simulink model "RL_sus_quarter_sim"  (R2025a)
settings: Solver=FixedStepAuto  StartTime=0.0  StopTime=20  FixedStep=0.001  RelTol=1e-3
model workspace (MAT data in the model file):
  G0 : Simulink.Parameter (value not decoded)
  Q_F : Simulink.Parameter (value not decoded)
  Q_dot_s : Simulink.Parameter (value not decoded)
  Q_dot_s_h : Simulink.Parameter (value not decoded)
  Q_dot_u : Simulink.Parameter (value not decoded)
  Q_flec : Simulink.Parameter (value not decoded)
  Q_flec_t : Simulink.Parameter (value not decoded)
  b_deflec : Simulink.Parameter (value not decoded)
  bump_height : Simulink.Parameter (value not decoded)
  bump_lenth : Simulink.Parameter (value not decoded)
  bump_start : Simulink.Parameter (value not decoded)
  f0 : Simulink.Parameter (value not decoded)
  kt : Simulink.Parameter (value not decoded)
  ms : Simulink.Parameter (value not decoded)
  n0 : Simulink.Parameter (value not decoded)
  n1 : Simulink.Parameter (value not decoded)
  omega_1 : Simulink.Parameter (value not decoded)
  omega_2 : Simulink.Parameter (value not decoded)
  omega_3 : Simulink.Parameter (value not decoded)
  omega_4 : Simulink.Parameter (value not decoded)
  ramp_height : Simulink.Parameter (value not decoded)
  ramp_lenth : Simulink.Parameter (value not decoded)
  ramp_start : Simulink.Parameter (value not decoded)
  sine_amp : Simulink.Parameter (value not decoded)
  sine_freq : Simulink.Parameter (value not decoded)
  u : Simulink.Parameter (value not decoded)
symbols that are objects in the model workspace (value not decoded): b_deflec, bump_height, bump_lenth, bump_start, f0, G0, kt, ms, n0, n1, omega_1, omega_2, omega_3, omega_4, Q_dot_s, Q_dot_s_h, Q_F, Q_flec, Q_flec_t, ramp_height, ramp_lenth, ramp_start, sine_amp, sine_freq
undefined symbols (not defined in the file): Ground, Hook, SH_ADD_new_as_as_xdef
libraries: fl_lib x250, nesl_utility x48, sharedTrackingLibrary x34, dspstat3 x18, simulink x3, deeplib x2, slpidlib x1
(part 9 of 12)

== system RL_sus_quarter_sim/Quarter_sys/Control/Y_1/Freq_imp/Low_with_Alpha/Subsystem/p1_k5 ==
  Translational Inerter : fl_lib/Mechanical/Translational Elements/Translational Inerter  B=1 kg  v_specify=off  v_priority=High  v=0 m/s  v_nominal_specify=off  v_nominal_value=1  v_nominal_unit=m/s  f_specify=off  f_priority=None  f=0 N  f_nominal_specify=off  f_nominal_value=1  f_nominal_unit=N
      settings: InternalSimscapePortConfiguration="{\"Bottom\":[],\"Left\":[{\"id\":\"R\",\"label\":\"R\",\"type\":\"foundation.mechanical.translational.translational\"}],\"Right\":[{\"id\":\"C\",\"label\":\"C\",\"type\":\"foundation.mechanical.translational.translational\"}],\"Top\":[]}"
  Translational Damper : fl_lib/Mechanical/Translational Elements/Translational Damper  D=2000 N*s/m  v_specify=off  v_priority=None  v=0 m/s  v_nominal_specify=off  v_nominal_value=1  v_nominal_unit=m/s  f_specify=off  f_priority=None  f=0 N  f_nominal_specify=off  f_nominal_value=1  f_nominal_unit=N
  Translational Spring1 : fl_lib/Mechanical/Translational Elements/Translational Spring  spr_rate=20000 N/m  v_specify=off  v_priority=None  v=0 m/s  v_nominal_specify=off  v_nominal_value=1  v_nominal_unit=m/s  f_specify=off  f_priority=None  f=0 N  f_nominal_specify=off  f_nominal_value=1  f_nominal_unit=N  x_specify=off  x_priority=High  x=0 m  x_nominal_specify=off  x_nominal_value=1  x_nominal_unit=m
  Conn1 : PMIOPort  Side=Right
  Conn2 : PMIOPort  Port=2  Side=Left
  connections:
  Translational Damper/LConn1 -- Conn2/RConn1 -- Translational Inerter/LConn1
  Translational Damper/RConn1 -- Translational Spring1/LConn1 -- Translational Inerter/RConn1
  Translational Spring1/RConn1 -- Conn1/RConn1

== system RL_sus_quarter_sim/Quarter_sys/Control/Y_1/Freq_imp/Low_with_Alpha/Subsystem/passive ==
  Translational Damper : fl_lib/Mechanical/Translational Elements/Translational Damper  D=2000 N*s/m  v_specify=off  v_priority=None  v=0 m/s  v_nominal_specify=off  v_nominal_value=1  v_nominal_unit=m/s  f_specify=off  f_priority=None  f=0 N  f_nominal_specify=off  f_nominal_value=1  f_nominal_unit=N
  Translational Spring1 : fl_lib/Mechanical/Translational Elements/Translational Spring  spr_rate=200000 N/m  v_specify=off  v_priority=None  v=0 m/s  v_nominal_specify=off  v_nominal_value=1  v_nominal_unit=m/s  f_specify=off  f_priority=None  f=0 N  f_nominal_specify=off  f_nominal_value=1  f_nominal_unit=N  x_specify=off  x_priority=High  x=0 m  x_nominal_specify=off  x_nominal_value=1  x_nominal_unit=m
  Conn1 : PMIOPort  Side=Right
  Conn2 : PMIOPort  Port=2  Side=Left
  connections:
  Translational Damper/RConn1 -- Translational Spring1/RConn1 -- Conn1/RConn1
  Conn2/RConn1 -- Translational Damper/LConn1 -- Translational Spring1/LConn1

== system RL_sus_quarter_sim/Quarter_sys/Control/Y_1/Freq_imp/high_with_Alpha/Subsystem/p1_k1 ==
  Translational Inerter : fl_lib/Mechanical/Translational Elements/Translational Inerter  B=1 kg  v_specify=off  v_priority=High  v=0 m/s  v_nominal_specify=off  v_nominal_value=1  v_nominal_unit=m/s  f_specify=off  f_priority=None  f=0 N  f_nominal_specify=off  f_nominal_value=1  f_nominal_unit=N
      settings: InternalSimscapePortConfiguration="{\"Bottom\":[],\"Left\":[{\"id\":\"R\",\"label\":\"R\",\"type\":\"foundation.mechanical.translational.translational\"}],\"Right\":[{\"id\":\"C\",\"label\":\"C\",\"type\":\"foundation.mechanical.translational.translational\"}],\"Top\":[]}"
  Translational Damper : fl_lib/Mechanical/Translational Elements/Translational Damper  D=2000 N*s/m  v_specify=off  v_priority=None  v=0 m/s  v_nominal_specify=off  v_nominal_value=1  v_nominal_unit=m/s  f_specify=off  f_priority=None  f=0 N  f_nominal_specify=off  f_nominal_value=1  f_nominal_unit=N
  Translational Spring1 : fl_lib/Mechanical/Translational Elements/Translational Spring  spr_rate=20000 N/m  v_specify=off  v_priority=None  v=0 m/s  v_nominal_specify=off  v_nominal_value=1  v_nominal_unit=m/s  f_specify=off  f_priority=None  f=0 N  f_nominal_specify=off  f_nominal_value=1  f_nominal_unit=N  x_specify=off  x_priority=High  x=0 m  x_nominal_specify=off  x_nominal_value=1  x_nominal_unit=m
  Conn1 : PMIOPort  Side=Right
  Conn2 : PMIOPort  Port=2  Side=Left
  connections:
  Conn1/RConn1 -- Translational Damper/RConn1 -- Translational Spring1/RConn1
  Translational Spring1/LConn1 -- Translational Inerter/RConn1
  Conn2/RConn1 -- Translational Damper/LConn1 -- Translational Inerter/LConn1

== system RL_sus_quarter_sim/Quarter_sys/Control/Y_1/Freq_imp/high_with_Alpha/Subsystem/p1_k2 ==
  Translational Inerter : fl_lib/Mechanical/Translational Elements/Translational Inerter  B=1 kg  v_specify=off  v_priority=High  v=0 m/s  v_nominal_specify=off  v_nominal_value=1  v_nominal_unit=m/s  f_specify=off  f_priority=None  f=0 N  f_nominal_specify=off  f_nominal_value=1  f_nominal_unit=N
      settings: InternalSimscapePortConfiguration="{\"Bottom\":[],\"Left\":[{\"id\":\"R\",\"label\":\"R\",\"type\":\"foundation.mechanical.translational.translational\"}],\"Right\":[{\"id\":\"C\",\"label\":\"C\",\"type\":\"foundation.mechanical.translational.translational\"}],\"Top\":[]}"
  Translational Damper : fl_lib/Mechanical/Translational Elements/Translational Damper  D=2000 N*s/m  v_specify=off  v_priority=None  v=0 m/s  v_nominal_specify=off  v_nominal_value=1  v_nominal_unit=m/s  f_specify=off  f_priority=None  f=0 N  f_nominal_specify=off  f_nominal_value=1  f_nominal_unit=N
  Translational Spring1 : fl_lib/Mechanical/Translational Elements/Translational Spring  spr_rate=20000 N/m  v_specify=off  v_priority=None  v=0 m/s  v_nominal_specify=off  v_nominal_value=1  v_nominal_unit=m/s  f_specify=off  f_priority=None  f=0 N  f_nominal_specify=off  f_nominal_value=1  f_nominal_unit=N  x_specify=off  x_priority=High  x=0 m  x_nominal_specify=off  x_nominal_value=1  x_nominal_unit=m
  Conn1 : PMIOPort  Side=Right
  Conn2 : PMIOPort  Port=2  Side=Left
  connections:
  Translational Inerter/LConn1 -- Translational Damper/LConn1 -- Conn2/RConn1
  Translational Spring1/RConn1 -- Translational Inerter/RConn1 -- Conn1/RConn1
  Translational Spring1/LConn1 -- Translational Damper/RConn1

== system RL_sus_quarter_sim/Quarter_sys/Control/Y_1/Freq_imp/high_with_Alpha/Subsystem/p1_k3 ==
  Translational Inerter : fl_lib/Mechanical/Translational Elements/Translational Inerter  B=1 kg  v_specify=off  v_priority=High  v=0 m/s  v_nominal_specify=off  v_nominal_value=1  v_nominal_unit=m/s  f_specify=off  f_priority=None  f=0 N  f_nominal_specify=off  f_nominal_value=1  f_nominal_unit=N
      settings: InternalSimscapePortConfiguration="{\"Bottom\":[],\"Left\":[{\"id\":\"R\",\"label\":\"R\",\"type\":\"foundation.mechanical.translational.translational\"}],\"Right\":[{\"id\":\"C\",\"label\":\"C\",\"type\":\"foundation.mechanical.translational.translational\"}],\"Top\":[]}"
  Translational Damper : fl_lib/Mechanical/Translational Elements/Translational Damper  D=2000 N*s/m  v_specify=off  v_priority=None  v=0 m/s  v_nominal_specify=off  v_nominal_value=1  v_nominal_unit=m/s  f_specify=off  f_priority=None  f=0 N  f_nominal_specify=off  f_nominal_value=1  f_nominal_unit=N
  Translational Spring1 : fl_lib/Mechanical/Translational Elements/Translational Spring  spr_rate=20000 N/m  v_specify=off  v_priority=None  v=0 m/s  v_nominal_specify=off  v_nominal_value=1  v_nominal_unit=m/s  f_specify=off  f_priority=None  f=0 N  f_nominal_specify=off  f_nominal_value=1  f_nominal_unit=N  x_specify=off  x_priority=High  x=0 m  x_nominal_specify=off  x_nominal_value=1  x_nominal_unit=m
  Conn1 : PMIOPort  Side=Right
  Conn2 : PMIOPort  Port=2  Side=Left
  connections:
  Conn2/RConn1 -- Translational Damper/LConn1 -- Translational Inerter/LConn1 -- Translational Spring1/LConn1
  Translational Inerter/RConn1 -- Conn1/RConn1 -- Translational Damper/RConn1 -- Translational Spring1/RConn1

== system RL_sus_quarter_sim/Quarter_sys/Control/Y_1/Freq_imp/high_with_Alpha/Subsystem/p1_k5 ==
  Translational Inerter : fl_lib/Mechanical/Translational Elements/Translational Inerter  B=1 kg  v_specify=off  v_priority=High  v=0 m/s  v_nominal_specify=off  v_nominal_value=1  v_nominal_unit=m/s  f_specify=off  f_priority=None  f=0 N  f_nominal_specify=off  f_nominal_value=1  f_nominal_unit=N
      settings: InternalSimscapePortConfiguration="{\"Bottom\":[],\"Left\":[{\"id\":\"R\",\"label\":\"R\",\"type\":\"foundation.mechanical.translational.translational\"}],\"Right\":[{\"id\":\"C\",\"label\":\"C\",\"type\":\"foundation.mechanical.translational.translational\"}],\"Top\":[]}"
  Translational Damper : fl_lib/Mechanical/Translational Elements/Translational Damper  D=2000 N*s/m  v_specify=off  v_priority=None  v=0 m/s  v_nominal_specify=off  v_nominal_value=1  v_nominal_unit=m/s  f_specify=off  f_priority=None  f=0 N  f_nominal_specify=off  f_nominal_value=1  f_nominal_unit=N
  Translational Spring1 : fl_lib/Mechanical/Translational Elements/Translational Spring  spr_rate=20000 N/m  v_specify=off  v_priority=None  v=0 m/s  v_nominal_specify=off  v_nominal_value=1  v_nominal_unit=m/s  f_specify=off  f_priority=None  f=0 N  f_nominal_specify=off  f_nominal_value=1  f_nominal_unit=N  x_specify=off  x_priority=High  x=0 m  x_nominal_specify=off  x_nominal_value=1  x_nominal_unit=m
  Conn1 : PMIOPort  Side=Right
  Conn2 : PMIOPort  Port=2  Side=Left
  connections:
  Translational Spring1/RConn1 -- Conn1/RConn1
  Translational Inerter/RConn1 -- Translational Spring1/LConn1 -- Translational Damper/RConn1
  Translational Inerter/LConn1 -- Conn2/RConn1 -- Translational Damper/LConn1

== system RL_sus_quarter_sim/Quarter_sys/Control/Y_1/Freq_imp/high_with_Alpha/Subsystem/passive ==
  Translational Damper : fl_lib/Mechanical/Translational Elements/Translational Damper  D=2000 N*s/m  v_specify=off  v_priority=None  v=0 m/s  v_nominal_specify=off  v_nominal_value=1  v_nominal_unit=m/s  f_specify=off  f_priority=None  f=0 N  f_nominal_specify=off  f_nominal_value=1  f_nominal_unit=N
  Translational Spring1 : fl_lib/Mechanical/Translational Elements/Translational Spring  spr_rate=200000 N/m  v_specify=off  v_priority=None  v=0 m/s  v_nominal_specify=off  v_nominal_value=1  v_nominal_unit=m/s  f_specify=off  f_priority=None  f=0 N  f_nominal_specify=off  f_nominal_value=1  f_nominal_unit=N  x_specify=off  x_priority=High  x=0 m  x_nominal_specify=off  x_nominal_value=1  x_nominal_unit=m
  Conn1 : PMIOPort  Side=Right
  Conn2 : PMIOPort  Port=2  Side=Left
  connections:
  Translational Spring1/LConn1 -- Translational Damper/LConn1 -- Conn2/RConn1
  Conn1/RConn1 -- Translational Spring1/RConn1 -- Translational Damper/RConn1

== system RL_sus_quarter_sim/Quarter_sys/Control/Y_1/Freq_imp1/Low_with_Alpha/Subsystem/p1_k1 ==
  Translational Inerter : fl_lib/Mechanical/Translational Elements/Translational Inerter  B=1 kg  v_specify=off  v_priority=High  v=0 m/s  v_nominal_specify=off  v_nominal_value=1  v_nominal_unit=m/s  f_specify=off  f_priority=None  f=0 N  f_nominal_specify=off  f_nominal_value=1  f_nominal_unit=N
      settings: InternalSimscapePortConfiguration="{\"Bottom\":[],\"Left\":[{\"id\":\"R\",\"label\":\"R\",\"type\":\"foundation.mechanical.translational.translational\"}],\"Right\":[{\"id\":\"C\",\"label\":\"C\",\"type\":\"foundation.mechanical.translational.translational\"}],\"Top\":[]}"
  Translational Damper : fl_lib/Mechanical/Translational Elements/Translational Damper  D=2000 N*s/m  v_specify=off  v_priority=None  v=0 m/s  v_nominal_specify=off  v_nominal_value=1  v_nominal_unit=m/s  f_specify=off  f_priority=None  f=0 N  f_nominal_specify=off  f_nominal_value=1  f_nominal_unit=N
  Translational Spring1 : fl_lib/Mechanical/Translational Elements/Translational Spring  spr_rate=20000 N/m  v_specify=off  v_priority=None  v=0 m/s  v_nominal_specify=off  v_nominal_value=1  v_nominal_unit=m/s  f_specify=off  f_priority=None  f=0 N  f_nominal_specify=off  f_nominal_value=1  f_nominal_unit=N  x_specify=off  x_priority=High  x=0 m  x_nominal_specify=off  x_nominal_value=1  x_nominal_unit=m
  Conn1 : PMIOPort  Side=Right
  Conn2 : PMIOPort  Port=2  Side=Left
  connections:
  Conn1/RConn1 -- Translational Damper/RConn1 -- Translational Spring1/RConn1
  Translational Spring1/LConn1 -- Translational Inerter/RConn1
  Conn2/RConn1 -- Translational Damper/LConn1 -- Translational Inerter/LConn1

== system RL_sus_quarter_sim/Quarter_sys/Control/Y_1/Freq_imp1/Low_with_Alpha/Subsystem/p1_k2 ==
  Translational Inerter : fl_lib/Mechanical/Translational Elements/Translational Inerter  B=1 kg  v_specify=off  v_priority=High  v=0 m/s  v_nominal_specify=off  v_nominal_value=1  v_nominal_unit=m/s  f_specify=off  f_priority=None  f=0 N  f_nominal_specify=off  f_nominal_value=1  f_nominal_unit=N
      settings: InternalSimscapePortConfiguration="{\"Bottom\":[],\"Left\":[{\"id\":\"R\",\"label\":\"R\",\"type\":\"foundation.mechanical.translational.translational\"}],\"Right\":[{\"id\":\"C\",\"label\":\"C\",\"type\":\"foundation.mechanical.translational.translational\"}],\"Top\":[]}"
  Translational Damper : fl_lib/Mechanical/Translational Elements/Translational Damper  D=2000 N*s/m  v_specify=off  v_priority=None  v=0 m/s  v_nominal_specify=off  v_nominal_value=1  v_nominal_unit=m/s  f_specify=off  f_priority=None  f=0 N  f_nominal_specify=off  f_nominal_value=1  f_nominal_unit=N
  Translational Spring1 : fl_lib/Mechanical/Translational Elements/Translational Spring  spr_rate=20000 N/m  v_specify=off  v_priority=None  v=0 m/s  v_nominal_specify=off  v_nominal_value=1  v_nominal_unit=m/s  f_specify=off  f_priority=None  f=0 N  f_nominal_specify=off  f_nominal_value=1  f_nominal_unit=N  x_specify=off  x_priority=High  x=0 m  x_nominal_specify=off  x_nominal_value=1  x_nominal_unit=m
  Conn1 : PMIOPort  Side=Right
  Conn2 : PMIOPort  Port=2  Side=Left
  connections:
  Translational Inerter/LConn1 -- Translational Damper/LConn1 -- Conn2/RConn1
  Translational Spring1/RConn1 -- Translational Inerter/RConn1 -- Conn1/RConn1
  Translational Spring1/LConn1 -- Translational Damper/RConn1

== system RL_sus_quarter_sim/Quarter_sys/Control/Y_1/Freq_imp1/Low_with_Alpha/Subsystem/p1_k3 ==
  Translational Inerter : fl_lib/Mechanical/Translational Elements/Translational Inerter  B=1 kg  v_specify=off  v_priority=High  v=0 m/s  v_nominal_specify=off  v_nominal_value=1  v_nominal_unit=m/s  f_specify=off  f_priority=None  f=0 N  f_nominal_specify=off  f_nominal_value=1  f_nominal_unit=N
      settings: InternalSimscapePortConfiguration="{\"Bottom\":[],\"Left\":[{\"id\":\"R\",\"label\":\"R\",\"type\":\"foundation.mechanical.translational.translational\"}],\"Right\":[{\"id\":\"C\",\"label\":\"C\",\"type\":\"foundation.mechanical.translational.translational\"}],\"Top\":[]}"
  Translational Damper : fl_lib/Mechanical/Translational Elements/Translational Damper  D=2000 N*s/m  v_specify=off  v_priority=None  v=0 m/s  v_nominal_specify=off  v_nominal_value=1  v_nominal_unit=m/s  f_specify=off  f_priority=None  f=0 N  f_nominal_specify=off  f_nominal_value=1  f_nominal_unit=N
  Translational Spring1 : fl_lib/Mechanical/Translational Elements/Translational Spring  spr_rate=20000 N/m  v_specify=off  v_priority=None  v=0 m/s  v_nominal_specify=off  v_nominal_value=1  v_nominal_unit=m/s  f_specify=off  f_priority=None  f=0 N  f_nominal_specify=off  f_nominal_value=1  f_nominal_unit=N  x_specify=off  x_priority=High  x=0 m  x_nominal_specify=off  x_nominal_value=1  x_nominal_unit=m
  Conn1 : PMIOPort  Side=Right
  Conn2 : PMIOPort  Port=2  Side=Left
  connections:
  Conn2/RConn1 -- Translational Damper/LConn1 -- Translational Inerter/LConn1 -- Translational Spring1/LConn1
  Translational Inerter/RConn1 -- Conn1/RConn1 -- Translational Damper/RConn1 -- Translational Spring1/RConn1

== system RL_sus_quarter_sim/Quarter_sys/Control/Y_1/Freq_imp1/Low_with_Alpha/Subsystem/p1_k5 ==
  Translational Inerter : fl_lib/Mechanical/Translational Elements/Translational Inerter  B=1 kg  v_specify=off  v_priority=High  v=0 m/s  v_nominal_specify=off  v_nominal_value=1  v_nominal_unit=m/s  f_specify=off  f_priority=None  f=0 N  f_nominal_specify=off  f_nominal_value=1  f_nominal_unit=N
      settings: InternalSimscapePortConfiguration="{\"Bottom\":[],\"Left\":[{\"id\":\"R\",\"label\":\"R\",\"type\":\"foundation.mechanical.translational.translational\"}],\"Right\":[{\"id\":\"C\",\"label\":\"C\",\"type\":\"foundation.mechanical.translational.translational\"}],\"Top\":[]}"
  Translational Damper : fl_lib/Mechanical/Translational Elements/Translational Damper  D=2000 N*s/m  v_specify=off  v_priority=None  v=0 m/s  v_nominal_specify=off  v_nominal_value=1  v_nominal_unit=m/s  f_specify=off  f_priority=None  f=0 N  f_nominal_specify=off  f_nominal_value=1  f_nominal_unit=N
  Translational Spring1 : fl_lib/Mechanical/Translational Elements/Translational Spring  spr_rate=20000 N/m  v_specify=off  v_priority=None  v=0 m/s  v_nominal_specify=off  v_nominal_value=1  v_nominal_unit=m/s  f_specify=off  f_priority=None  f=0 N  f_nominal_specify=off  f_nominal_value=1  f_nominal_unit=N  x_specify=off  x_priority=High  x=0 m  x_nominal_specify=off  x_nominal_value=1  x_nominal_unit=m
  Conn1 : PMIOPort  Side=Right
  Conn2 : PMIOPort  Port=2  Side=Left
  connections:
  Translational Spring1/RConn1 -- Conn1/RConn1
  Translational Inerter/RConn1 -- Translational Spring1/LConn1 -- Translational Damper/RConn1
  Translational Inerter/LConn1 -- Conn2/RConn1 -- Translational Damper/LConn1

== system RL_sus_quarter_sim/Quarter_sys/Control/Y_1/Freq_imp1/Low_with_Alpha/Subsystem/passive ==
  Translational Damper : fl_lib/Mechanical/Translational Elements/Translational Damper  D=2000 N*s/m  v_specify=off  v_priority=None  v=0 m/s  v_nominal_specify=off  v_nominal_value=1  v_nominal_unit=m/s  f_specify=off  f_priority=None  f=0 N  f_nominal_specify=off  f_nominal_value=1  f_nominal_unit=N
  Translational Spring1 : fl_lib/Mechanical/Translational Elements/Translational Spring  spr_rate=200000 N/m  v_specify=off  v_priority=None  v=0 m/s  v_nominal_specify=off  v_nominal_value=1  v_nominal_unit=m/s  f_specify=off  f_priority=None  f=0 N  f_nominal_specify=off  f_nominal_value=1  f_nominal_unit=N  x_specify=off  x_priority=High  x=0 m  x_nominal_specify=off  x_nominal_value=1  x_nominal_unit=m
  Conn1 : PMIOPort  Side=Right
  Conn2 : PMIOPort  Port=2  Side=Left
  connections:
  Translational Spring1/LConn1 -- Translational Damper/LConn1 -- Conn2/RConn1
  Conn1/RConn1 -- Translational Spring1/RConn1 -- Translational Damper/RConn1

== system RL_sus_quarter_sim/Quarter_sys/Control/Y_1/Freq_imp1/high_with_Alpha/Subsystem/p1_k1 ==
  Translational Inerter : fl_lib/Mechanical/Translational Elements/Translational Inerter  B=1 kg  v_specify=off  v_priority=High  v=0 m/s  v_nominal_specify=off  v_nominal_value=1  v_nominal_unit=m/s  f_specify=off  f_priority=None  f=0 N  f_nominal_specify=off  f_nominal_value=1  f_nominal_unit=N
      settings: InternalSimscapePortConfiguration="{\"Bottom\":[],\"Left\":[{\"id\":\"R\",\"label\":\"R\",\"type\":\"foundation.mechanical.translational.translational\"}],\"Right\":[{\"id\":\"C\",\"label\":\"C\",\"type\":\"foundation.mechanical.translational.translational\"}],\"Top\":[]}"
  Translational Damper : fl_lib/Mechanical/Translational Elements/Translational Damper  D=2000 N*s/m  v_specify=off  v_priority=None  v=0 m/s  v_nominal_specify=off  v_nominal_value=1  v_nominal_unit=m/s  f_specify=off  f_priority=None  f=0 N  f_nominal_specify=off  f_nominal_value=1  f_nominal_unit=N
  Translational Spring1 : fl_lib/Mechanical/Translational Elements/Translational Spring  spr_rate=20000 N/m  v_specify=off  v_priority=None  v=0 m/s  v_nominal_specify=off  v_nominal_value=1  v_nominal_unit=m/s  f_specify=off  f_priority=None  f=0 N  f_nominal_specify=off  f_nominal_value=1  f_nominal_unit=N  x_specify=off  x_priority=High  x=0 m  x_nominal_specify=off  x_nominal_value=1  x_nominal_unit=m
  Conn1 : PMIOPort  Side=Right
  Conn2 : PMIOPort  Port=2  Side=Left
  connections:
  Translational Inerter/LConn1 -- Translational Damper/LConn1 -- Conn2/RConn1
  Translational Spring1/LConn1 -- Translational Inerter/RConn1
  Translational Spring1/RConn1 -- Translational Damper/RConn1 -- Conn1/RConn1

== system RL_sus_quarter_sim/Quarter_sys/Control/Y_1/Freq_imp1/high_with_Alpha/Subsystem/p1_k2 ==
  Translational Inerter : fl_lib/Mechanical/Translational Elements/Translational Inerter  B=1 kg  v_specify=off  v_priority=High  v=0 m/s  v_nominal_specify=off  v_nominal_value=1  v_nominal_unit=m/s  f_specify=off  f_priority=None  f=0 N  f_nominal_specify=off  f_nominal_value=1  f_nominal_unit=N
      settings: InternalSimscapePortConfiguration="{\"Bottom\":[],\"Left\":[{\"id\":\"R\",\"label\":\"R\",\"type\":\"foundation.mechanical.translational.translational\"}],\"Right\":[{\"id\":\"C\",\"label\":\"C\",\"type\":\"foundation.mechanical.translational.translational\"}],\"Top\":[]}"
  Translational Damper : fl_lib/Mechanical/Translational Elements/Translational Damper  D=2000 N*s/m  v_specify=off  v_priority=None  v=0 m/s  v_nominal_specify=off  v_nominal_value=1  v_nominal_unit=m/s  f_specify=off  f_priority=None  f=0 N  f_nominal_specify=off  f_nominal_value=1  f_nominal_unit=N
  Translational Spring1 : fl_lib/Mechanical/Translational Elements/Translational Spring  spr_rate=20000 N/m  v_specify=off  v_priority=None  v=0 m/s  v_nominal_specify=off  v_nominal_value=1  v_nominal_unit=m/s  f_specify=off  f_priority=None  f=0 N  f_nominal_specify=off  f_nominal_value=1  f_nominal_unit=N  x_specify=off  x_priority=High  x=0 m  x_nominal_specify=off  x_nominal_value=1  x_nominal_unit=m
  Conn1 : PMIOPort  Side=Right
  Conn2 : PMIOPort  Port=2  Side=Left
  connections:
  Translational Spring1/LConn1 -- Translational Damper/RConn1
  Conn1/RConn1 -- Translational Inerter/RConn1 -- Translational Spring1/RConn1
  Conn2/RConn1 -- Translational Damper/LConn1 -- Translational Inerter/LConn1

== system RL_sus_quarter_sim/Quarter_sys/Control/Y_1/Freq_imp1/high_with_Alpha/Subsystem/p1_k3 ==
  Translational Inerter : fl_lib/Mechanical/Translational Elements/Translational Inerter  B=1 kg  v_specify=off  v_priority=High  v=0 m/s  v_nominal_specify=off  v_nominal_value=1  v_nominal_unit=m/s  f_specify=off  f_priority=None  f=0 N  f_nominal_specify=off  f_nominal_value=1  f_nominal_unit=N
      settings: InternalSimscapePortConfiguration="{\"Bottom\":[],\"Left\":[{\"id\":\"R\",\"label\":\"R\",\"type\":\"foundation.mechanical.translational.translational\"}],\"Right\":[{\"id\":\"C\",\"label\":\"C\",\"type\":\"foundation.mechanical.translational.translational\"}],\"Top\":[]}"
  Translational Damper : fl_lib/Mechanical/Translational Elements/Translational Damper  D=2000 N*s/m  v_specify=off  v_priority=None  v=0 m/s  v_nominal_specify=off  v_nominal_value=1  v_nominal_unit=m/s  f_specify=off  f_priority=None  f=0 N  f_nominal_specify=off  f_nominal_value=1  f_nominal_unit=N
  Translational Spring1 : fl_lib/Mechanical/Translational Elements/Translational Spring  spr_rate=20000 N/m  v_specify=off  v_priority=None  v=0 m/s  v_nominal_specify=off  v_nominal_value=1  v_nominal_unit=m/s  f_specify=off  f_priority=None  f=0 N  f_nominal_specify=off  f_nominal_value=1  f_nominal_unit=N  x_specify=off  x_priority=High  x=0 m  x_nominal_specify=off  x_nominal_value=1  x_nominal_unit=m
  Conn1 : PMIOPort  Side=Right
  Conn2 : PMIOPort  Port=2  Side=Left
  connections:
  Translational Spring1/RConn1 -- Translational Damper/RConn1 -- Conn1/RConn1 -- Translational Inerter/RConn1
  Translational Spring1/LConn1 -- Translational Inerter/LConn1 -- Translational Damper/LConn1 -- Conn2/RConn1

== system RL_sus_quarter_sim/Quarter_sys/Control/Y_1/Freq_imp1/high_with_Alpha/Subsystem/p1_k5 ==
  Translational Inerter : fl_lib/Mechanical/Translational Elements/Translational Inerter  B=1 kg  v_specify=off  v_priority=High  v=0 m/s  v_nominal_specify=off  v_nominal_value=1  v_nominal_unit=m/s  f_specify=off  f_priority=None  f=0 N  f_nominal_specify=off  f_nominal_value=1  f_nominal_unit=N
      settings: InternalSimscapePortConfiguration="{\"Bottom\":[],\"Left\":[{\"id\":\"R\",\"label\":\"R\",\"type\":\"foundation.mechanical.translational.translational\"}],\"Right\":[{\"id\":\"C\",\"label\":\"C\",\"type\":\"foundation.mechanical.translational.translational\"}],\"Top\":[]}"
  Translational Damper : fl_lib/Mechanical/Translational Elements/Translational Damper  D=2000 N*s/m  v_specify=off  v_priority=None  v=0 m/s  v_nominal_specify=off  v_nominal_value=1  v_nominal_unit=m/s  f_specify=off  f_priority=None  f=0 N  f_nominal_specify=off  f_nominal_value=1  f_nominal_unit=N
  Translational Spring1 : fl_lib/Mechanical/Translational Elements/Translational Spring  spr_rate=20000 N/m  v_specify=off  v_priority=None  v=0 m/s  v_nominal_specify=off  v_nominal_value=1  v_nominal_unit=m/s  f_specify=off  f_priority=None  f=0 N  f_nominal_specify=off  f_nominal_value=1  f_nominal_unit=N  x_specify=off  x_priority=High  x=0 m  x_nominal_specify=off  x_nominal_value=1  x_nominal_unit=m
  Conn1 : PMIOPort  Side=Right
  Conn2 : PMIOPort  Port=2  Side=Left
  connections:
  Translational Damper/LConn1 -- Conn2/RConn1 -- Translational Inerter/LConn1
  Translational Damper/RConn1 -- Translational Spring1/LConn1 -- Translational Inerter/RConn1
  Translational Spring1/RConn1 -- Conn1/RConn1

== system RL_sus_quarter_sim/Quarter_sys/Control/Y_1/Freq_imp1/high_with_Alpha/Subsystem/passive ==
  Translational Damper : fl_lib/Mechanical/Translational Elements/Translational Damper  D=2000 N*s/m  v_specify=off  v_priority=None  v=0 m/s  v_nominal_specify=off  v_nominal_value=1  v_nominal_unit=m/s  f_specify=off  f_priority=None  f=0 N  f_nominal_specify=off  f_nominal_value=1  f_nominal_unit=N
  Translational Spring1 : fl_lib/Mechanical/Translational Elements/Translational Spring  spr_rate=200000 N/m  v_specify=off  v_priority=None  v=0 m/s  v_nominal_specify=off  v_nominal_value=1  v_nominal_unit=m/s  f_specify=off  f_priority=None  f=0 N  f_nominal_specify=off  f_nominal_value=1  f_nominal_unit=N  x_specify=off  x_priority=High  x=0 m  x_nominal_specify=off  x_nominal_value=1  x_nominal_unit=m
  Conn1 : PMIOPort  Side=Right
  Conn2 : PMIOPort  Port=2  Side=Left
  connections:
  Translational Damper/RConn1 -- Translational Spring1/RConn1 -- Conn1/RConn1
  Conn2/RConn1 -- Translational Damper/LConn1 -- Translational Spring1/LConn1

== system RL_sus_quarter_sim/Quarter_sys/Control/Y_1/IFEKF FDC/Subsystem/MATLAB Function2/EKF epsilon ==
  y : Inport
  epsilon : Inport  Port=2
  Constant : Constant  Value=diag([0,0,1,0])
  Constant7 : Constant  Value=500  SampleTime=0.001
  Extended Kalman Filter1 : sharedTrackingLibrary/Extended Kalman Filter  StateTransitionFcn=IFEKF_tfcn_ep  HasStateTransitionJacobianFcn=on  StateTransitionJacobianFcn=IFEKF_jcob_fcn_ep  HasAdditiveProcessNoise=Additive  ProcessNoise=[0,0,1e-7,1e-10]  HasTimeVaryingProcessNoise=on  HasStateTransitionFcnExtraArgument=1  InitialState=[0;-0.2;1*2*pi;0.2;]  InitialStateCovariance=[1e-1,1e-1,1e-1,1e-5]  MeasurementFcn1=IFEKF_measure_fcn_mod  HasMeasurementJacobianFcn1=on  MeasurementJacobianFcn1=IFEKF_mea_jcob_fcn_mod  HasMeasurementEnablePort1=off  HasAdditiveMeasurementNoise1=Additive  MeasurementNoise1=0.0001  HasTimeVaryingMeasurementNoise1=on  HasMeasurementFcnExtraArgument1=0  HasMeasurementWrapping1=off  MeasurementFcn2=myMeasurementFcn  HasMeasurementJacobianFcn2=off  HasMeasurementEnablePort2=off  HasAdditiveMeasurementNoise2=Additive  MeasurementNoise2=1  HasTimeVaryingMeasurementNoise2=off  HasMeasurementFcnExtraArgument2=0  HasMeasurementWrapping2=off  MeasurementFcn3=myMeasurementFcn  HasMeasurementJacobianFcn3=off  HasMeasurementEnablePort3=off  HasAdditiveMeasurementNoise3=Additive  MeasurementNoise3=1  HasTimeVaryingMeasurementNoise3=off  HasMeasurementFcnExtraArgument3=0  HasMeasurementWrapping3=off  MeasurementFcn4=myMeasurementFcn  HasMeasurementJacobianFcn4=off  HasMeasurementEnablePort4=off  HasAdditiveMeasurementNoise4=Additive  MeasurementNoise4=1  HasTimeVaryingMeasurementNoise4=off  HasMeasurementFcnExtraArgument4=0  HasMeasurementWrapping4=off  MeasurementFcn5=myMeasurementFcn  HasMeasurementJacobianFcn5=off  HasMeasurementEnablePort5=off  HasAdditiveMeasurementNoise5=Additive  MeasurementNoise5=1  HasTimeVaryingMeasurementNoise5=off  HasMeasurementFcnExtraArgument5=0  HasMeasurementWrapping5=off  EnableMultirate=off  StateTransitionFcnSampleTime=1  MeasurementFcn1SampleTime=1  MeasurementFcn2SampleTime=1  MeasurementFcn3SampleTime=1  MeasurementFcn4SampleTime=1  MeasurementFcn5SampleTime=1  UseCurrentEstimator=off  OutputStateCovariance=on  DataType=double  SampleTime=0.001  NumberOfMeasurements=1
  Gain6 : Gain  Gain=1/2/pi
  Scope6 : Scope
      settings: ActiveDisplayYMinimum=-0.3996  ActiveDisplayYMaximum=6.53697  DataLoggingVariableName=ScopeData2
  Selector1 : Selector  InputPortWidth=4  IndexOptions=Index vector (dialog)  Indices=[1]  OutputSizes=1
  Selector8 : Selector  InputPortWidth=4  IndexOptions=Index vector (dialog)  Indices=[3]  OutputSizes=1
  x1hat : Outport
  P : Outport  Port=2
  debug : Outport  Port=3
  xhat_pred : Outport  Port=4
  y_residual : Outport  Port=5
  omega : Outport  Port=6
  wires:
  y/1 -> Extended Kalman Filter1/3
  Extended Kalman Filter1/2 -> P/1
  Constant7/1 -> Extended Kalman Filter1/4
  epsilon/1 -> Extended Kalman Filter1/2
  Constant/1 -> Extended Kalman Filter1/1
  Gain6/1 -> omega/1, Scope6/1
  Selector8/1 -> Gain6/1
  Extended Kalman Filter1/1 -> Selector1/1, Selector8/1
  Selector1/1 -> x1hat/1

== system RL_sus_quarter_sim/Quarter_sys/Control/Y_1/IFEKF FDC/Subsystem/MATLAB Function2/EKF simple Amp ==
  y : Inport
  epsilon : Inport  Port=2
  Constant5 : Constant  Value=0.1e-5
  Constant7 : Constant  Value=0.11  SampleTime=0.001
  Extended Kalman Filter1 : sharedTrackingLibrary/Extended Kalman Filter  StateTransitionFcn=IFEKF_tfcn_amp  HasStateTransitionJacobianFcn=on  StateTransitionJacobianFcn=IFEKF_jcob_fcn_amp  HasAdditiveProcessNoise=Additive  ProcessNoise=[0,0,1e-7,1e-10]  HasTimeVaryingProcessNoise=on  HasStateTransitionFcnExtraArgument=1  InitialState=[0;-0.5;2*pi;0.5;]  InitialStateCovariance=[1e-1,1e-1,1e-1,1e-5]  MeasurementFcn1=IFEKF_measure_fcn_amp  HasMeasurementJacobianFcn1=on  MeasurementJacobianFcn1=IFEKF_mea_jcob_fcn_amp  HasMeasurementEnablePort1=off  HasAdditiveMeasurementNoise1=Additive  MeasurementNoise1=0.0001  HasTimeVaryingMeasurementNoise1=on  HasMeasurementFcnExtraArgument1=0  HasMeasurementWrapping1=off  MeasurementFcn2=myMeasurementFcn  HasMeasurementJacobianFcn2=off  HasMeasurementEnablePort2=off  HasAdditiveMeasurementNoise2=Additive  MeasurementNoise2=1  HasTimeVaryingMeasurementNoise2=off  HasMeasurementFcnExtraArgument2=0  HasMeasurementWrapping2=off  MeasurementFcn3=myMeasurementFcn  HasMeasurementJacobianFcn3=off  HasMeasurementEnablePort3=off  HasAdditiveMeasurementNoise3=Additive  MeasurementNoise3=1  HasTimeVaryingMeasurementNoise3=off  HasMeasurementFcnExtraArgument3=0  HasMeasurementWrapping3=off  MeasurementFcn4=myMeasurementFcn  HasMeasurementJacobianFcn4=off  HasMeasurementEnablePort4=off  HasAdditiveMeasurementNoise4=Additive  MeasurementNoise4=1  HasTimeVaryingMeasurementNoise4=off  HasMeasurementFcnExtraArgument4=0  HasMeasurementWrapping4=off  MeasurementFcn5=myMeasurementFcn  HasMeasurementJacobianFcn5=off  HasMeasurementEnablePort5=off  HasAdditiveMeasurementNoise5=Additive  MeasurementNoise5=1  HasTimeVaryingMeasurementNoise5=off  HasMeasurementFcnExtraArgument5=0  HasMeasurementWrapping5=off  EnableMultirate=off  StateTransitionFcnSampleTime=1  MeasurementFcn1SampleTime=1  MeasurementFcn2SampleTime=1  MeasurementFcn3SampleTime=1  MeasurementFcn4SampleTime=1  MeasurementFcn5SampleTime=1  UseCurrentEstimator=off  OutputStateCovariance=on  DataType=double  SampleTime=0.001  NumberOfMeasurements=1
  Gain6 : Gain  Gain=1/2/pi
  MATLAB Function : MATLAB Function
  Scope1 : Scope
      settings: ActiveDisplayYMinimum=-1.3479  ActiveDisplayYMaximum=7.13108  DataLoggingVariableName=ScopeData7
  Scope6 : Scope
      settings: ActiveDisplayYMinimum=0.9999988  ActiveDisplayYMaximum=1.0000001
  Selector1 : Selector  InputPortWidth=4  IndexOptions=Index vector (dialog)  Indices=[1]  OutputSizes=1
  Selector8 : Selector  InputPortWidth=4  IndexOptions=Index vector (dialog)  Indices=[3]  OutputSizes=1
  x1hat : Outport
  P : Outport  Port=2
  debug : Outport  Port=3
  xhat_pred : Outport  Port=4
  y_residual : Outport  Port=5
  omega : Outport  Port=6
  wires:
  epsilon/1 -> Extended Kalman Filter1/2
  Constant7/1 -> Extended Kalman Filter1/4
  Constant5/1 -> MATLAB Function/1(gamma)
  Extended Kalman Filter1/2 -> P/1
  y/1 -> Extended Kalman Filter1/3
  MATLAB Function/1(y) -> Extended Kalman Filter1/1
  Extended Kalman Filter1/1 -> Selector1/1, Selector8/1, Scope1/1
  Selector8/1 -> Gain6/1
  Gain6/1 -> omega/1, Scope6/1
  Selector1/1 -> x1hat/1

== system RL_sus_quarter_sim/Quarter_sys/Control/Y_1/IFEKF FDC/Subsystem/MATLAB Function2/IFEKF simple ==
  y : Inport
  Constant : Constant  Value=diag([0,0,0,0,1])
  Constant7 : Constant  Value=10  SampleTime=0.001
  Extended Kalman Filter1 : sharedTrackingLibrary/Extended Kalman Filter  StateTransitionFcn=IFEKF_tfcn_simp  HasStateTransitionJacobianFcn=on  StateTransitionJacobianFcn=IFEKF_jcob_fcn_simp  HasAdditiveProcessNoise=Additive  ProcessNoise=[0,0,1e-7,1e-10,0]  HasTimeVaryingProcessNoise=on  HasStateTransitionFcnExtraArgument=0  InitialState=[0;-1;0;-1;0.1*pi;]  InitialStateCovariance=[1e-1,1e-1,1e-1,1e-1,1e-5]  MeasurementFcn1=IFEKF_measure_fcn_simp  HasMeasurementJacobianFcn1=on  MeasurementJacobianFcn1=IFEKF_mea_jcob_fcn_simp  HasMeasurementEnablePort1=off  HasAdditiveMeasurementNoise1=Additive  MeasurementNoise1=0.0001  HasTimeVaryingMeasurementNoise1=on  HasMeasurementFcnExtraArgument1=0  HasMeasurementWrapping1=off  MeasurementFcn2=myMeasurementFcn  HasMeasurementJacobianFcn2=off  HasMeasurementEnablePort2=off  HasAdditiveMeasurementNoise2=Additive  MeasurementNoise2=1  HasTimeVaryingMeasurementNoise2=off  HasMeasurementFcnExtraArgument2=0  HasMeasurementWrapping2=off  MeasurementFcn3=myMeasurementFcn  HasMeasurementJacobianFcn3=off  HasMeasurementEnablePort3=off  HasAdditiveMeasurementNoise3=Additive  MeasurementNoise3=1  HasTimeVaryingMeasurementNoise3=off  HasMeasurementFcnExtraArgument3=0  HasMeasurementWrapping3=off  MeasurementFcn4=myMeasurementFcn  HasMeasurementJacobianFcn4=off  HasMeasurementEnablePort4=off  HasAdditiveMeasurementNoise4=Additive  MeasurementNoise4=1  HasTimeVaryingMeasurementNoise4=off  HasMeasurementFcnExtraArgument4=0  HasMeasurementWrapping4=off  MeasurementFcn5=myMeasurementFcn  HasMeasurementJacobianFcn5=off  HasMeasurementEnablePort5=off  HasAdditiveMeasurementNoise5=Additive  MeasurementNoise5=1  HasTimeVaryingMeasurementNoise5=off  HasMeasurementFcnExtraArgument5=0  HasMeasurementWrapping5=off  EnableMultirate=off  StateTransitionFcnSampleTime=1  MeasurementFcn1SampleTime=1  MeasurementFcn2SampleTime=1  MeasurementFcn3SampleTime=1  MeasurementFcn4SampleTime=1  MeasurementFcn5SampleTime=1  UseCurrentEstimator=off  OutputStateCovariance=on  DataType=double  SampleTime=0.001  NumberOfMeasurements=1
  Gain6 : Gain  Gain=1/2/pi
  Scope1 : Scope
      settings: ActiveDisplayYMinimum=-108223.31295  ActiveDisplayYMaximum=120159.3313  DataLoggingVariableName=ScopeData2
  Scope6 : Scope
      settings: ActiveDisplayYMinimum=-5.04517  ActiveDisplayYMaximum=3.95687  DataLoggingVariableName=ScopeData3
  Selector1 : Selector  InputPortWidth=5  IndexOptions=Index vector (dialog)  Indices=[1]  OutputSizes=1
  Selector8 : Selector  InputPortWidth=5  IndexOptions=Index vector (dialog)  Indices=[5]  OutputSizes=1
  x1hat : Outport
  P : Outport  Port=2
  debug : Outport  Port=3
  xhat_pred : Outport  Port=4
  y_residual : Outport  Port=5
  omega : Outport  Port=6
  wires:
  y/1 -> Extended Kalman Filter1/2
  Extended Kalman Filter1/2 -> P/1
  Constant7/1 -> Extended Kalman Filter1/3
  Constant/1 -> Extended Kalman Filter1/1
  Gain6/1 -> omega/1, Scope6/1
  Selector8/1 -> Gain6/1
  Selector1/1 -> x1hat/1
  Extended Kalman Filter1/1 -> Selector1/1, Selector8/1, Scope1/1

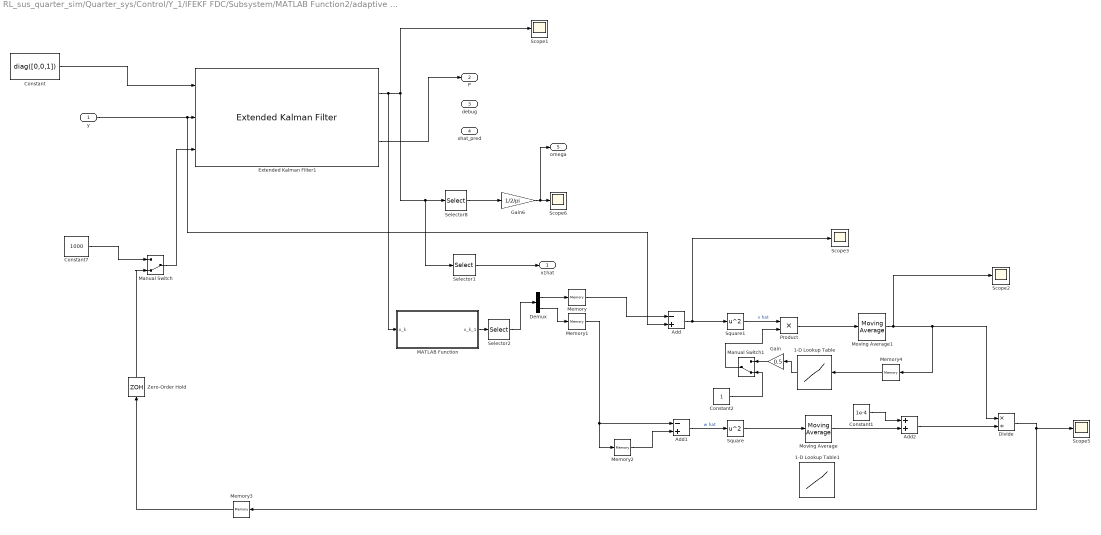
== system RL_sus_quarter_sim/Quarter_sys/Control/Y_1/IFEKF FDC/Subsystem/MATLAB Function2/adaptive IFEKF sdimple_3 ==
  y : Inport
  1-D Lookup Table : Lookup_n-D  NumberOfTableDimensions=1  BreakpointsForDimension1=[0;0.050000000000000003;0.070000000000000007;0.10000000000000001;0.5;3;5;50]  BeginIndexSearchUsingPreviousIndexResult=on  Table=[1;0.5;0.3;0.2;0.1;0.1;0.1;0.1]  InterpMethod=Nearest  InternalRulePriority=Speed  RndMeth=Simplest
  1-D Lookup Table1 : Lookup_n-D  NumberOfTableDimensions=1  BreakpointsForDimension1=[0;0.5;1;2;3;5;10;20;50]  BeginIndexSearchUsingPreviousIndexResult=on  Table=[1;0.9;0.8;0.8;0.8;0.5;0.4;0.3;0.3]  InterpMethod=Nearest  InternalRulePriority=Speed  RndMeth=Simplest
  Add : Sum  Inputs=-+
  Add1 : Sum  Inputs=-+
  Add2 : Sum
  Constant : Constant  Value=diag([0,0,1])
  Constant1 : Constant  Value=1e-4
  Constant2 : Constant
  Constant7 : Constant  Value=1000  SampleTime=0.001
  Demux : Demux  Outputs=2
  Divide : Product  Inputs=*/
  Extended Kalman Filter1 : sharedTrackingLibrary/Extended Kalman Filter  StateTransitionFcn=IFEKF_tfcn_simp_3  HasStateTransitionJacobianFcn=on  StateTransitionJacobianFcn=IFEKF_jcob_fcn_simp_3  HasAdditiveProcessNoise=Additive  ProcessNoise=[1e-7,1e-10,0]  HasTimeVaryingProcessNoise=on  HasStateTransitionFcnExtraArgument=0  InitialState=[0;-1;10*2*pi;]  InitialStateCovariance=[1e-1,1e-1,1e-5]  MeasurementFcn1=IFEKF_measure_fcn_simp_3  HasMeasurementJacobianFcn1=on  MeasurementJacobianFcn1=IFEKF_mea_jcob_fcn_simp_3  HasMeasurementEnablePort1=off  HasAdditiveMeasurementNoise1=Additive  MeasurementNoise1=0.0001  HasTimeVaryingMeasurementNoise1=on  HasMeasurementFcnExtraArgument1=0  HasMeasurementWrapping1=off  MeasurementFcn2=myMeasurementFcn  HasMeasurementJacobianFcn2=off  HasMeasurementEnablePort2=off  HasAdditiveMeasurementNoise2=Additive  MeasurementNoise2=1  HasTimeVaryingMeasurementNoise2=off  HasMeasurementFcnExtraArgument2=0  HasMeasurementWrapping2=off  MeasurementFcn3=myMeasurementFcn  HasMeasurementJacobianFcn3=off  HasMeasurementEnablePort3=off  HasAdditiveMeasurementNoise3=Additive  MeasurementNoise3=1  HasTimeVaryingMeasurementNoise3=off  HasMeasurementFcnExtraArgument3=0  HasMeasurementWrapping3=off  MeasurementFcn4=myMeasurementFcn  HasMeasurementJacobianFcn4=off  HasMeasurementEnablePort4=off  HasAdditiveMeasurementNoise4=Additive  MeasurementNoise4=1  HasTimeVaryingMeasurementNoise4=off  HasMeasurementFcnExtraArgument4=0  HasMeasurementWrapping4=off  MeasurementFcn5=myMeasurementFcn  HasMeasurementJacobianFcn5=off  HasMeasurementEnablePort5=off  HasAdditiveMeasurementNoise5=Additive  MeasurementNoise5=1  HasTimeVaryingMeasurementNoise5=off  HasMeasurementFcnExtraArgument5=0  HasMeasurementWrapping5=off  EnableMultirate=off  StateTransitionFcnSampleTime=1  MeasurementFcn1SampleTime=1  MeasurementFcn2SampleTime=1  MeasurementFcn3SampleTime=1  MeasurementFcn4SampleTime=1  MeasurementFcn5SampleTime=1  UseCurrentEstimator=off  OutputStateCovariance=on  DataType=double  SampleTime=0.001  NumberOfMeasurements=1
  Gain : Gain  Gain=0.5
  Gain6 : Gain  Gain=1/2/pi
  MATLAB Function : MATLAB Function  TreatAsAtomicUnit=on
  Manual Switch : ManualSwitch  CurrentSetting=0
  Manual Switch1 : ManualSwitch  CurrentSetting=0
  Memory : Memory  InitialCondition=5
  Memory1 : Memory
  Memory2 : Memory  InitialCondition=1
  Memory3 : Memory  InitialCondition=10
  Memory4 : Memory
  Moving Average : dspstat3/Moving Average  Method=Exponential weighting  ForgettingFactorPort=off  SpecifyWindowLength=off  WindowLength=100  OverlapLength=50  AllowArbitraryInputLength=on  ForgettingFactor=0.999  SimulateUsing=Interpreted execution
  Moving Average1 : dspstat3/Moving Average  Method=Exponential weighting  ForgettingFactorPort=off  SpecifyWindowLength=off  WindowLength=100  OverlapLength=50  AllowArbitraryInputLength=on  ForgettingFactor=0.999  SimulateUsing=Interpreted execution
  Product : Product
  Scope{1..3,5..6} (5 alike) : Scope
      Scope1 settings: ActiveDisplayYMinimum=-1.53674  ActiveDisplayYMaximum=3.8307  DataLoggingVariableName=ScopeData2
      Scope2 settings: ActiveDisplayYMinimum=-3.12038  ActiveDisplayYMaximum=28.12449
      Scope3 settings: ActiveDisplayYMinimum=-6.54945  ActiveDisplayYMaximum=6.61329  DataLoggingVariableName=ScopeData5
      Scope5 settings: ActiveDisplayYMinimum=-0.41328  ActiveDisplayYMaximum=0.25655  DataLoggingVariableName=ScopeData7
      Scope6 settings: ActiveDisplayYMinimum=8.52023  ActiveDisplayYMaximum=10.23596
  Selector1 : Selector  InputPortWidth=3  IndexOptions=Index vector (dialog)  Indices=[1]  OutputSizes=1
  Selector2 : Selector  InputPortWidth=3  IndexOptions=Index vector (dialog)  Indices=[1 3]  OutputSizes=1
  Selector8 : Selector  InputPortWidth=3  IndexOptions=Index vector (dialog)  Indices=[3]  OutputSizes=1
  Square : Math  Operator=square
  Square1 : Math  Operator=square
  Zero-Order Hold : ZeroOrderHold  SampleTime=0.001
  x1hat : Outport
  P : Outport  Port=2
  debug : Outport  Port=3
  xhat_pred : Outport  Port=4
  omega : Outport  Port=5
  wires:
  Constant2/1 -> Manual Switch1/2
  Manual Switch1/1 -> Product/2
  Memory4/1 -> 1-D Lookup Table/1
  1-D Lookup Table/1 -> Gain/1
  Moving Average1/1 -> Divide/1, Memory4/1, Scope2/1
  Product/1 -> Moving Average1/1
  Constant1/1 -> Add2/1
  Add2/1 -> Divide/2
  Zero-Order Hold/1 -> Manual Switch/2
  y/1 -> Extended Kalman Filter1/2, Add/2
  Memory3/1 -> Zero-Order Hold/1
  Manual Switch/1 -> Extended Kalman Filter1/3
  Divide/1 -> Scope5/1, Memory3/1
  Moving Average/1 -> Add2/2
  Square1/1 -> Product/1  "v hat"
  Square/1 -> Moving Average/1
  Add1/1 -> Square/1  "w hat"
  Add/1 -> Square1/1, Scope3/1
  Memory2/1 -> Add1/2
  Memory1/1 -> Memory2/1, Add1/1
  Demux/2 -> Memory1/1
  Demux/1 -> Memory/1
  Selector2/1 -> Demux/1
  Extended Kalman Filter1/2 -> P/1
  Gain6/1 -> omega/1, Scope6/1
  MATLAB Function/1(x_k_1) -> Selector2/1
  Extended Kalman Filter1/1 -> Selector1/1, Selector8/1, Scope1/1, MATLAB Function/1(x_k)
  Selector1/1 -> x1hat/1
  Constant/1 -> Extended Kalman Filter1/1
  Constant7/1 -> Manual Switch/1
  Selector8/1 -> Gain6/1
  Memory/1 -> Add/1
  Gain/1 -> Manual Switch1/1
